simulink model "buck4ph_switching"  (R2024a)
settings: Solver=ode1  StartTime=0.0  StopTime=0.001  FixedStep=2e-08  RelTol=1e-3
undefined symbols (not defined in the file): load_end_a, load_start_a, slew_a_per_us, step_trigger_s, temp_c, vin_v
settings Model: Creator=ejliixa  LastModifiedBy=ejliixa

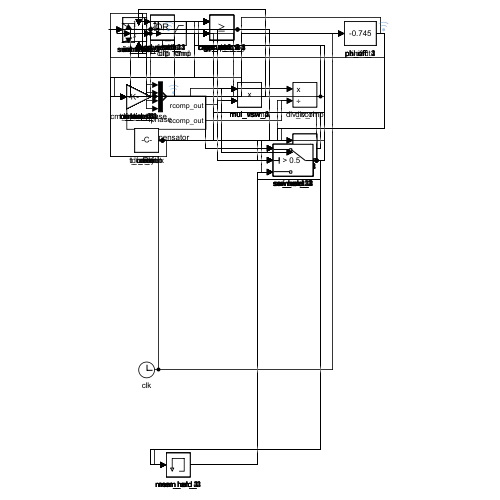
[thumbnail: Simulink's stored preview of the top-level diagram]
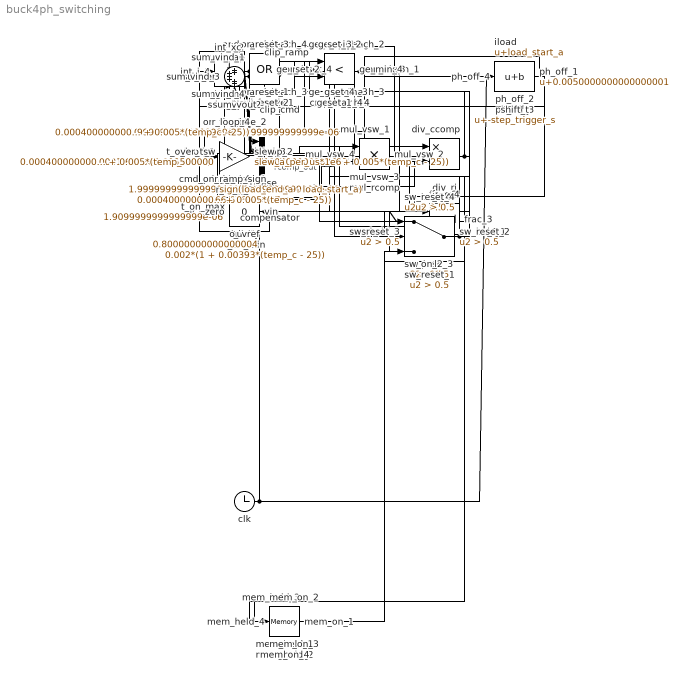
== system buck4ph_switching ==
  Ri : Constant  Value=0.002*(1 + 0.00393*(temp_c - 25))
  and_hi : Logic  AllPortsSameDT=off  OutDataTypeStr=boolean
  and_lo : Logic  AllPortsSameDT=off  OutDataTypeStr=boolean
  and_reach_{1..4} (4 alike) : Logic  AllPortsSameDT=off  OutDataTypeStr=boolean
  clip_cmd : Saturate  UpperLimit=300  LowerLimit=0
  clip_ramp : Saturate  UpperLimit=abs(load_end_a - load_start_a)  LowerLimit=0
  clk : Clock
  cmd_per_phase : Gain  Gain=0.25
  cmp_err_neg : RelationalOperator  Operator=<  OutDataTypeStr=boolean  RndMeth=Simplest  InputSameDT=off
  cmp_err_pos : RelationalOperator  Operator=>  OutDataTypeStr=boolean  RndMeth=Simplest  InputSameDT=off
  cmp_hi : RelationalOperator  Operator=>  OutDataTypeStr=boolean  RndMeth=Simplest  InputSameDT=off
  cmp_lo : RelationalOperator  Operator=<  OutDataTypeStr=boolean  RndMeth=Simplest  InputSameDT=off
  cmp_reach_{1..4} (4 alike) : RelationalOperator  OutDataTypeStr=boolean  RndMeth=Simplest  InputSameDT=off
  compensator : Subsystem
  div_ccomp : Product  Inputs=*/
  div_ri : Product  Inputs=*/
  dt_const : Constant  Value=2e-08
  esr : Gain  Gain=0.00014999999999999999
  frac_{1..4} (4 alike) : Math  Operator=mod
  freeze : Switch  Criteria=u2 > Threshold  Threshold=0.5  SaturateOnIntegerOverflow=off  InputSameDT=off
  ge_max_{1..4} (4 alike) : RelationalOperator  OutDataTypeStr=boolean  RndMeth=Simplest  InputSameDT=off
  ge_min_{1..4} (4 alike) : RelationalOperator  OutDataTypeStr=boolean  RndMeth=Simplest  InputSameDT=off
  gm : Gain  Gain=0.00020000000000000001
  i_limit : Constant  Value=300
  i_total : Sum  Inputs=++++
  iload : Bias  Bias=load_start_a  SaturateOnIntegerOverflow=off
  int_i_{1..4} (4 alike) : Integrator  InitialCondition=load_start_a/4
  int_vc : Integrator  InitialCondition=0.80000000000000004
  int_xc : Integrator  InitialCondition=load_start_a*(0.002*(1 + 0.00393*(temp_c - 25)))
  inv_cout : Gain  Gain=166.66666666666666
  inv_l_{1..4} (4 alike) : Gain  Gain=6666666.666666667
  iphase : Mux
  mem_held_{1..4} (4 alike) : Memory  InitialCondition=load_start_a/4
  mem_on_{1..4} (4 alike) : Memory
  mul_rcomp : Product
  mul_vsw_{1..4} (4 alike) : Product
  on_time_{1..4} (4 alike) : Gain  Gain=1.9999999999999999e-06
  one : Constant
  or_freeze : Logic  Operator=OR  AllPortsSameDT=off  OutDataTypeStr=boolean
  or_reset_{1..4} (4 alike) : Logic  Operator=OR  AllPortsSameDT=off  OutDataTypeStr=boolean
  ph_off_1 : Bias  Bias=0.0050000000000000001  SaturateOnIntegerOverflow=off
  ph_off_2 : Bias  Bias=-0.245  SaturateOnIntegerOverflow=off
  ph_off_3 : Bias  Bias=-0.495  SaturateOnIntegerOverflow=off
  ph_off_4 : Bias  Bias=-0.745  SaturateOnIntegerOverflow=off
  r_loop_{1..4} (4 alike) : Gain  Gain=0.00040000000000000002*(1 + 0.00393*(temp_c - 25)) + 0.0011999999999999999*(1 + 0.005*(temp_c - 25))
  ramp_sign : Gain  Gain=sign(load_end_a - load_start_a)
  set_{1..4} (4 alike) : RelationalOperator  Operator=<  OutDataTypeStr=boolean  RndMeth=Simplest  InputSameDT=off
  shift_t : Bias  Bias=-step_trigger_s  SaturateOnIntegerOverflow=off
  slew : Gain  Gain=slew_a_per_us*1e6
  sum_cap : Sum  Inputs=+-
  sum_comp : Sum
  sum_err : Sum  Inputs=+-
  sum_vind_{1..4} (4 alike) : Sum  Inputs=+--
  sum_vout : Sum
  sw_held_{1..4} (4 alike) : Switch  Criteria=u2 > Threshold  Threshold=0.5  SaturateOnIntegerOverflow=off  InputSameDT=off
  sw_on_{1..4} (4 alike) : Switch  Criteria=u2 > Threshold  Threshold=0.5  SaturateOnIntegerOverflow=off  InputSameDT=off
  sw_reset_{1..4} (4 alike) : Switch  Criteria=u2 > Threshold  Threshold=0.5  SaturateOnIntegerOverflow=off  InputSameDT=off
  t_on_max : Constant  Value=1.9099999999999999e-06
  t_on_min : Constant  Value=2e-08
  t_over_tsw : Gain  Gain=500000
  unity : Constant
  vin : Constant  Value=vin_v
  vref : Constant  Value=0.80000000000000004
  zero : Constant  Value=0
  wires:
  clk/1 -> shift_t/1, t_over_tsw/1
  shift_t/1 -> slew/1
  slew/1 -> clip_ramp/1
  clip_ramp/1 -> ramp_sign/1
  ramp_sign/1 -> iload/1
  vref/1 -> sum_err/1
  sum_vout/1 -> sum_err/2, sum_vind_1/2, sum_vind_2/2, sum_vind_3/2, sum_vind_4/2
  sum_err/1 -> gm/1, cmp_err_pos/1, cmp_err_neg/1
  gm/1 -> mul_rcomp/1, div_ccomp/1
  compensator/1(rcomp_out) -> mul_rcomp/2
  compensator/2(ccomp_out) -> div_ccomp/2
  div_ccomp/1 -> freeze/3
  zero/1 -> freeze/1, cmp_lo/2, cmp_err_pos/2, cmp_err_neg/2, sw_reset_1/1, sw_reset_2/1, sw_reset_3/1, sw_reset_4/1
  or_freeze/1 -> freeze/2
  freeze/1 -> int_xc/1
  int_xc/1 -> sum_comp/1
  mul_rcomp/1 -> sum_comp/2
  sum_comp/1 -> div_ri/1
  Ri/1 -> div_ri/2
  div_ri/1 -> clip_cmd/1, cmp_hi/1, cmp_lo/1
  i_limit/1 -> cmp_hi/2
  cmp_hi/1 -> and_hi/1
  cmp_err_pos/1 -> and_hi/2
  cmp_lo/1 -> and_lo/1
  cmp_err_neg/1 -> and_lo/2
  and_hi/1 -> or_freeze/1
  and_lo/1 -> or_freeze/2
  clip_cmd/1 -> cmd_per_phase/1
  i_total/1 -> sum_cap/1
  iload/1 -> sum_cap/2
  sum_cap/1 -> inv_cout/1, esr/1
  inv_cout/1 -> int_vc/1
  esr/1 -> sum_vout/1
  int_vc/1 -> sum_vout/2
  t_over_tsw/1 -> ph_off_1/1, ph_off_2/1, ph_off_3/1, ph_off_4/1
  ph_off_1/1 -> frac_1/1
  unity/1 -> frac_1/2, frac_2/2, frac_3/2, frac_4/2
  frac_1/1 -> on_time_1/1
  on_time_1/1 -> set_1/1, ge_min_1/1, ge_max_1/1
  dt_const/1 -> set_1/2, set_2/2, set_3/2, set_4/2
  t_on_min/1 -> ge_min_1/2, ge_min_2/2, ge_min_3/2, ge_min_4/2
  t_on_max/1 -> ge_max_1/2, ge_max_2/2, ge_max_3/2, ge_max_4/2
  cmd_per_phase/1 -> sw_held_1/1, sw_held_2/1, sw_held_3/1, sw_held_4/1
  set_1/1 -> sw_held_1/2, sw_on_1/2
  mem_held_1/1 -> sw_held_1/3
  sw_held_1/1 -> mem_held_1/1, cmp_reach_1/2
  int_i_1/1 -> cmp_reach_1/1, r_loop_1/1, i_total/1, iphase/1
  cmp_reach_1/1 -> and_reach_1/1
  ge_min_1/1 -> and_reach_1/2
  and_reach_1/1 -> or_reset_1/1
  ge_max_1/1 -> or_reset_1/2
  or_reset_1/1 -> sw_reset_1/2
  mem_on_1/1 -> sw_reset_1/3
  one/1 -> sw_on_1/1, sw_on_2/1, sw_on_3/1, sw_on_4/1
  sw_reset_1/1 -> sw_on_1/3
  sw_on_1/1 -> mem_on_1/1, mul_vsw_1/1
  vin/1 -> mul_vsw_1/2, mul_vsw_2/2, mul_vsw_3/2, mul_vsw_4/2
  mul_vsw_1/1 -> sum_vind_1/1
  r_loop_1/1 -> sum_vind_1/3
  sum_vind_1/1 -> inv_l_1/1
  inv_l_1/1 -> int_i_1/1
  ph_off_2/1 -> frac_2/1
  frac_2/1 -> on_time_2/1
  on_time_2/1 -> set_2/1, ge_min_2/1, ge_max_2/1
  set_2/1 -> sw_held_2/2, sw_on_2/2
  mem_held_2/1 -> sw_held_2/3
  sw_held_2/1 -> mem_held_2/1, cmp_reach_2/2
  int_i_2/1 -> cmp_reach_2/1, r_loop_2/1, i_total/2, iphase/2
  cmp_reach_2/1 -> and_reach_2/1
  ge_min_2/1 -> and_reach_2/2
  and_reach_2/1 -> or_reset_2/1
  ge_max_2/1 -> or_reset_2/2
  or_reset_2/1 -> sw_reset_2/2
  mem_on_2/1 -> sw_reset_2/3
  sw_reset_2/1 -> sw_on_2/3
  sw_on_2/1 -> mem_on_2/1, mul_vsw_2/1
  mul_vsw_2/1 -> sum_vind_2/1
  r_loop_2/1 -> sum_vind_2/3
  sum_vind_2/1 -> inv_l_2/1
  inv_l_2/1 -> int_i_2/1
  ph_off_3/1 -> frac_3/1
  frac_3/1 -> on_time_3/1
  on_time_3/1 -> set_3/1, ge_min_3/1, ge_max_3/1
  set_3/1 -> sw_held_3/2, sw_on_3/2
  mem_held_3/1 -> sw_held_3/3
  sw_held_3/1 -> mem_held_3/1, cmp_reach_3/2
  int_i_3/1 -> cmp_reach_3/1, r_loop_3/1, i_total/3, iphase/3
  cmp_reach_3/1 -> and_reach_3/1
  ge_min_3/1 -> and_reach_3/2
  and_reach_3/1 -> or_reset_3/1
  ge_max_3/1 -> or_reset_3/2
  or_reset_3/1 -> sw_reset_3/2
  mem_on_3/1 -> sw_reset_3/3
  sw_reset_3/1 -> sw_on_3/3
  sw_on_3/1 -> mem_on_3/1, mul_vsw_3/1
  mul_vsw_3/1 -> sum_vind_3/1
  r_loop_3/1 -> sum_vind_3/3
  sum_vind_3/1 -> inv_l_3/1
  inv_l_3/1 -> int_i_3/1
  ph_off_4/1 -> frac_4/1
  frac_4/1 -> on_time_4/1
  on_time_4/1 -> set_4/1, ge_min_4/1, ge_max_4/1
  set_4/1 -> sw_held_4/2, sw_on_4/2
  mem_held_4/1 -> sw_held_4/3
  sw_held_4/1 -> mem_held_4/1, cmp_reach_4/2
  int_i_4/1 -> cmp_reach_4/1, r_loop_4/1, i_total/4, iphase/4
  cmp_reach_4/1 -> and_reach_4/1
  ge_min_4/1 -> and_reach_4/2
  and_reach_4/1 -> or_reset_4/1
  ge_max_4/1 -> or_reset_4/2
  or_reset_4/1 -> sw_reset_4/2
  mem_on_4/1 -> sw_reset_4/3
  sw_reset_4/1 -> sw_on_4/3
  sw_on_4/1 -> mem_on_4/1, mul_vsw_4/1
  mul_vsw_4/1 -> sum_vind_4/1
  r_loop_4/1 -> sum_vind_4/3
  sum_vind_4/1 -> inv_l_4/1
  inv_l_4/1 -> int_i_4/1

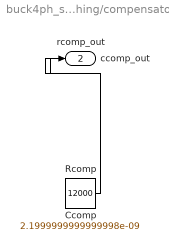
== system buck4ph_switching/compensator ==
  Ccomp : Constant  Value=2.1999999999999998e-09
  Rcomp : Constant  Value=12000
  rcomp_out : Outport
  ccomp_out : Outport  Port=2
  wires:
  Rcomp/1 -> rcomp_out/1
  Ccomp/1 -> ccomp_out/1
